simulink model "Symmetric"  (R2018a)
settings: Solver=VariableStepAuto  StartTime=0.0  StopTime=0.001  RelTol=1e-3
undefined symbols (not defined in the file or in its folder): fdesignblkfcn, G1, G2, G3, G4, G5, G6, G7, G8, gcbh, get, T
libraries: dspsrcs4 x1, dspxfrm3 x1, dspobslib x1
(part 1 of 2)
settings Model: Creator=Daniel  LastModifiedBy=Daniel

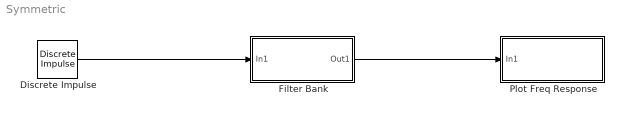
== system Symmetric ==
  Discrete Impulse : dspsrcs4/Discrete  Impulse  Delay=0  SampleTime=T  FrameSample=128  OutputFrames=off  dataType=double  isSigned=on  wordLen=16  udDataType=sfix(16)  fracBitsMode=Best precision  numFracBits=15  OutDataTypeStr=double  LastOutDataTypeStr=double
  "Filter Bank " : Subsystem
  Plot Freq Response : Subsystem
  wires:
  "Filter Bank "/1(Out1) -> Plot Freq Response/1(In1)
  Discrete Impulse/1 -> "Filter Bank "/1(In1)

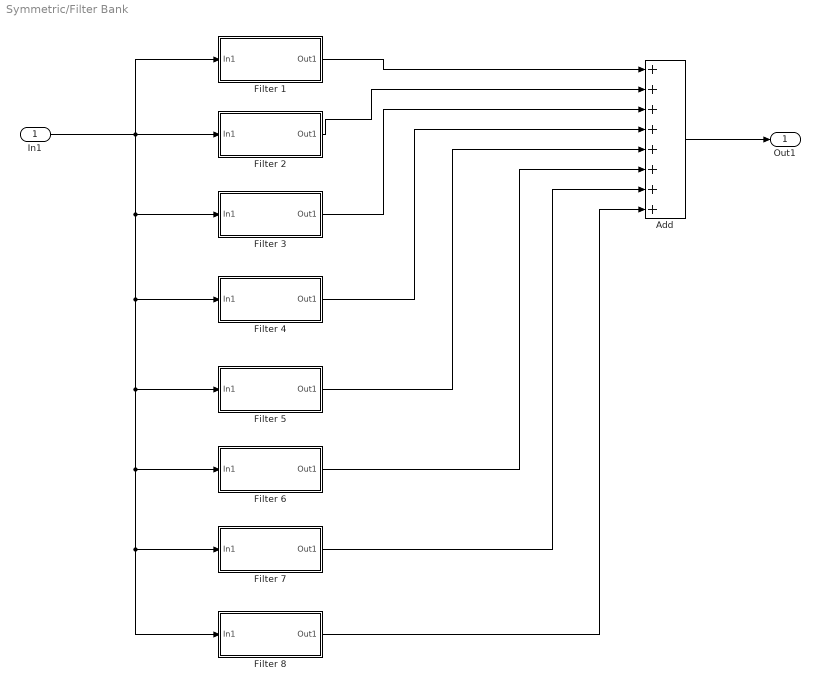
== system Symmetric/Filter Bank  ==
  In1 : Inport
  Add : Sum  Inputs=++++++++
  Filter 1 : Subsystem
  Filter 2 : Subsystem
  Filter 3 : Subsystem
  Filter 4 : Subsystem
  Filter 5 : Subsystem
  Filter 6 : Subsystem
  Filter 7 : Subsystem
  Filter 8 : Subsystem
  Out1 : Outport
  wires:
  In1/1 -> Filter 3/1(In1), Filter 6/1(In1), Filter 8/1(In1), Filter 7/1(In1), Filter 5/1(In1), Filter 4/1(In1), Filter 1/1(In1), Filter 2/1(In1)
  Add/1 -> Out1/1
  Filter 1/1(Out1) -> Add/1
  Filter 2/1(Out1) -> Add/2
  Filter 3/1(Out1) -> Add/3
  Filter 4/1(Out1) -> Add/4
  Filter 5/1(Out1) -> Add/5
  Filter 6/1(Out1) -> Add/6
  Filter 7/1(Out1) -> Add/7
  Filter 8/1(Out1) -> Add/8

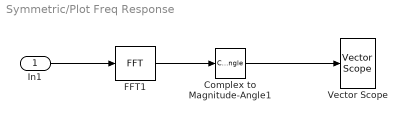
== system Symmetric/Plot Freq Response ==
  In1 : Inport
  Complex to Magnitude-Angle1 : ComplexToMagnitudeAngle  Output=Magnitude
  FFT1 : dspxfrm3/FFT  FFTImplementation=Auto  CompMethod=Table lookup  TableOpt=NEW  TableOptActive=Speed  BitRevOrder=off  Normalize=off  InheritFFTLength=on  FFTLength=64  WrapInput=on  roundingMode=Floor  overflowMode=off  firstCoeffDataTypeStr=Inherit: Same word length as input  firstCoeffLastDataTypeStr=Inherit: Same word length as input  outputMin=[]  outputMax=[]
  Vector Scope : dspobslib/Vector Scope  ScopeProperties=off  Domain=Frequency  HorizSpan=1  DisplayProperties=off  AxisGrid=on  Memory=off  FrameNumber=off  AxisLegend=off  AxisZoom=off  OpenScopeAtSimStart=on  OpenScopeImmediately=off  FigPos=get(0,'defaultfigureposition')  AxisProperties=on  XUnits=Hertz  XRange=[0...Fs/2]  InheritXIncr=on  XIncr=1  XLabel=Samples  XLimit=Auto  XMin=0  XMax=1  XStart=0  YUnits=dB  YLabel=|Magnitude (dB)|  LineProperties=off  XAxisParamsVer=6.9
      settings: SourceProductName=DSP System Toolbox  SourceProductBaseCode=DS  YMin=0.0723692553519949  YMax=69.3188381671759
  wires:
  In1/1 -> FFT1/1
  FFT1/1 -> Complex to Magnitude-Angle1/1
  Complex to Magnitude-Angle1/1 -> Vector Scope/1

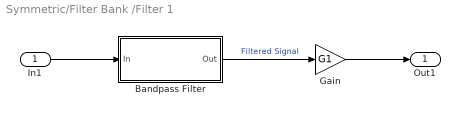
== system Symmetric/Filter Bank /Filter 1 ==
  In1 : Inport
  Bandpass Filter : Subsystem  DialogController=fdesignblkfcn  InitFcn=fdesignblkfcn(gcbh, {'InitFcn'});  mask(Bandpass Filter){}
      mask help: Design a bandpass filter
      settings: CopyFcn=fdesignblkfcn(gcbh, {'CopyFcn'});
      mask Help: helpview(mapfilelocation('dsp'), 'dspbandpassfilter');
      mask Display: disp('Bandpass');
  Gain : Gain  Gain=G1
  Out1 : Outport
  wires:
  Bandpass Filter/1(Out) -> Gain/1  "Filtered Signal"
  In1/1 -> Bandpass Filter/1(In)
  Gain/1 -> Out1/1

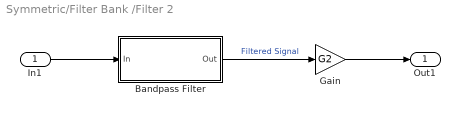
== system Symmetric/Filter Bank /Filter 2 ==
  In1 : Inport
  Bandpass Filter : Subsystem  DialogController=fdesignblkfcn  InitFcn=fdesignblkfcn(gcbh, {'InitFcn'});  mask(Bandpass Filter){}
      mask help: Design a bandpass filter
      settings: CopyFcn=fdesignblkfcn(gcbh, {'CopyFcn'});
      mask Help: helpview(mapfilelocation('dsp'), 'dspbandpassfilter');
      mask Display: disp('Bandpass');
  Gain : Gain  Gain=G2
  Out1 : Outport
  wires:
  Bandpass Filter/1(Out) -> Gain/1  "Filtered Signal"
  In1/1 -> Bandpass Filter/1(In)
  Gain/1 -> Out1/1

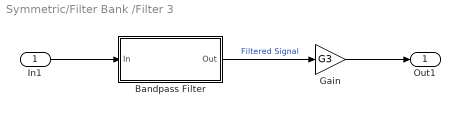
== system Symmetric/Filter Bank /Filter 3 ==
  In1 : Inport
  Bandpass Filter : Subsystem  DialogController=fdesignblkfcn  InitFcn=fdesignblkfcn(gcbh, {'InitFcn'});  mask(Bandpass Filter){}
      mask help: Design a bandpass filter
      settings: CopyFcn=fdesignblkfcn(gcbh, {'CopyFcn'});
      mask Help: helpview(mapfilelocation('dsp'), 'dspbandpassfilter');
      mask Display: disp('Bandpass');
  Gain : Gain  Gain=G3
  Out1 : Outport
  wires:
  Bandpass Filter/1(Out) -> Gain/1  "Filtered Signal"
  In1/1 -> Bandpass Filter/1(In)
  Gain/1 -> Out1/1

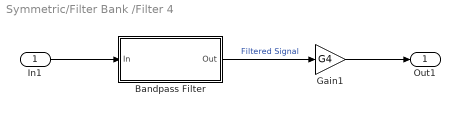
== system Symmetric/Filter Bank /Filter 4 ==
  In1 : Inport
  Bandpass Filter : Subsystem  DialogController=fdesignblkfcn  InitFcn=fdesignblkfcn(gcbh, {'InitFcn'});  mask(Bandpass Filter){}
      mask help: Design a bandpass filter
      settings: CopyFcn=fdesignblkfcn(gcbh, {'CopyFcn'});
      mask Help: helpview(mapfilelocation('dsp'), 'dspbandpassfilter');
      mask Display: disp('Bandpass');
  Gain1 : Gain  Gain=G4
  Out1 : Outport
  wires:
  Bandpass Filter/1(Out) -> Gain1/1  "Filtered Signal"
  In1/1 -> Bandpass Filter/1(In)
  Gain1/1 -> Out1/1

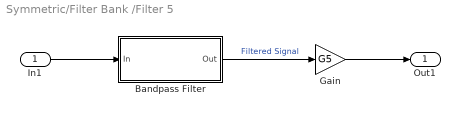
== system Symmetric/Filter Bank /Filter 5 ==
  In1 : Inport
  Bandpass Filter : Subsystem  DialogController=fdesignblkfcn  InitFcn=fdesignblkfcn(gcbh, {'InitFcn'});  mask(Bandpass Filter){}
      mask help: Design a bandpass filter
      settings: CopyFcn=fdesignblkfcn(gcbh, {'CopyFcn'});
      mask Help: helpview(mapfilelocation('dsp'), 'dspbandpassfilter');
      mask Display: disp('Bandpass');
  Gain : Gain  Gain=G5
  Out1 : Outport
  wires:
  Bandpass Filter/1(Out) -> Gain/1  "Filtered Signal"
  In1/1 -> Bandpass Filter/1(In)
  Gain/1 -> Out1/1

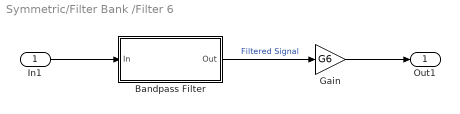
== system Symmetric/Filter Bank /Filter 6 ==
  In1 : Inport
  Bandpass Filter : Subsystem  DialogController=fdesignblkfcn  InitFcn=fdesignblkfcn(gcbh, {'InitFcn'});  mask(Bandpass Filter){}
      mask help: Design a bandpass filter
      settings: CopyFcn=fdesignblkfcn(gcbh, {'CopyFcn'});
      mask Help: helpview(mapfilelocation('dsp'), 'dspbandpassfilter');
      mask Display: disp('Bandpass');
  Gain : Gain  Gain=G6
  Out1 : Outport
  wires:
  Bandpass Filter/1(Out) -> Gain/1  "Filtered Signal"
  In1/1 -> Bandpass Filter/1(In)
  Gain/1 -> Out1/1

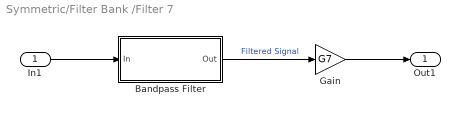
== system Symmetric/Filter Bank /Filter 7 ==
  In1 : Inport
  Bandpass Filter : Subsystem  DialogController=fdesignblkfcn  InitFcn=fdesignblkfcn(gcbh, {'InitFcn'});  mask(Bandpass Filter){}
      mask help: Design a bandpass filter
      settings: CopyFcn=fdesignblkfcn(gcbh, {'CopyFcn'});
      mask Help: helpview(mapfilelocation('dsp'), 'dspbandpassfilter');
      mask Display: disp('Bandpass');
  Gain : Gain  Gain=G7
  Out1 : Outport
  wires:
  Bandpass Filter/1(Out) -> Gain/1  "Filtered Signal"
  In1/1 -> Bandpass Filter/1(In)
  Gain/1 -> Out1/1

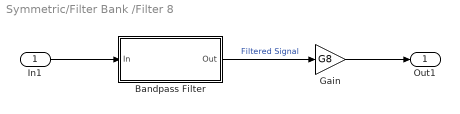
== system Symmetric/Filter Bank /Filter 8 ==
  In1 : Inport
  Bandpass Filter : Subsystem  DialogController=fdesignblkfcn  InitFcn=fdesignblkfcn(gcbh, {'InitFcn'});  mask(Bandpass Filter){}
      mask help: Design a bandpass filter
      settings: CopyFcn=fdesignblkfcn(gcbh, {'CopyFcn'});
      mask Help: helpview(mapfilelocation('dsp'), 'dspbandpassfilter');
      mask Display: disp('Bandpass');
  Gain : Gain  Gain=G8
  Out1 : Outport
  wires:
  Bandpass Filter/1(Out) -> Gain/1  "Filtered Signal"
  In1/1 -> Bandpass Filter/1(In)
  Gain/1 -> Out1/1

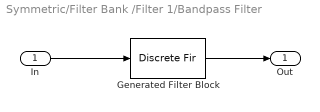
== system Symmetric/Filter Bank /Filter 1/Bandpass Filter ==
  In : Inport
  Generated Filter Block : DiscreteFir  Tag=BlockMethodSubSystem  Coefficients=[-0.288095935880251341 0.0525413418793297254 0.0469661528164785833 0.0413638961371985137 0.035743441875384814 0.0302610985045535484 0.0249161502944590801 0.0198560448668691492 0.0150617771881191003 0.010666253622455062 0.00662957256733126641 0.00307310029519767408 -7.12960758679805751e-05 -0.00269835686235154635 -0.00489597889786988483 -0.00657724977724275309 -0.00785309685969738311 -0.00864490861053823952 -0.00908979973506063472 -0.00911294285184072357 -0.00886997142217804853 -0.00828269872784345891 -0.00753185105272888202 -0.0065224375252314077 -0.0054576348610641005 -0.00422078667992279669 -0.00303593884382812084 -0.00174830873380574518 -0.000624644827463872749 0.000565354589150086689 0.00147289315421754116 0.00248164411845878258 0.00297649801950551803 0.00390644550655125378 0.00398986221425357869 0.00403163182400657384 0.00456913300373868771 0.00432952584417146263 0.00400413183887830121 0.00344452385152928036 0.00301759298676832367 0.0024648592619853733 0.00193704472346889608 0.00124269990373978298 0.000548146504904496691 -0.000233013280134805774 -0.000928086752325718274 -0.0016079036239721406 -0.00214342466057358509 -0.00261716452405418281 -0.00294642152557405852 -0.00321455590136646976 -0.00335513396218764222 -0.00343992999519496636 -0.00340818795304924848 -0.00331340319439810734 -0.00310534230123610776 -0.00283734411446902529 -0.0024686874963907833 -0.0020569757750758472 -0.00157932562542066851 -0.00108587602369365505 -0.00057464084255065865 -8.13931265320316902e-05 0.000379597218251630979 0.000803932237389910504 0.00116688807154375512 0.00140346382358171864 0.0017586610006951487 0.00174634027324323086 0.00186915640884384644 0.00190447992190369416 0.00184536222554758096 0.00164416184478038594 0.00144815028055871129 0.00120349413676317614 0.000953390304450837294 0.000615258083736531418 0.000258467885861202173 -0.000150488665692159111 -0.000520219390183063418 -0.000891696334957693291 -0.00120771657172187097 -0.00152010790567788136 -0.00177394667003233884 -0.00201259740633604042 -0.00217171226694658649 -0.00228852113553741935 -0.00230795208856010743 -0.00228053186210913725 -0.00215770975631921673 -0.00200597290924939579 -0.00178203504450490774 -0.00154713966436696108 -0.0012589304553587981 -0.000975184109959554841 -0.000647493809809341399 -0.000346389813347766965 -1.05485888533850436e-05 0.000256005081726213808 0.000577266056077218172 0.000756941456292188619 0.000985192320275318388 0.00113782558874355854 0.00118798764884436013 0.00123247243293567567 0.0012391642454049911 0.00116301132690384973 0.00103099208911635503 0.000863506020181792431 0.000681473816022045114 0.000453132507183181708 0.000193466705602888557 -0.000106363452799241865 -0.000406032554897162526 -0.000706800381284402863 -0.000984810227707108186 -0.00126094782477854201 -0.00150626261146827745 -0.00173150850840898709 -0.00190142474726660783 -0.00202931247623803742 -0.0020845945038517914 -0.00209873265242488871 -0.00204732530938491093 -0.00195812536072512014 -0.00181273083358852614 -0.00163528458599522986 -0.00140292268371900982 -0.00115138365696888963 -0.000853404855691656953 -0.000560408972579917513 -0.000237305797226729692 5.14958393311397135e-05 0.000346091011103256041 0.000621721693698512579 0.000829669047200214983 0.00105359212742192295 0.00120447865377228515 0.00129240756542236775 0.00134653604455318922 0.00134602513970211971 0.00127532081186506035 0.00113833590676117534 0.000964261511990258569 0.00074878023214015486 0.000496570402411653368 0.000204119261869774429 -0.000108583699207686528 -0.000434128584114584217 -0.000750409925752096568 -0.00106718699240494199 -0.00137092701931430219 -0.00166158721467703414 -0.00191329706170356413 -0.00212840560559363458 -0.00228636162366604306 -0.00239347382873119361 -0.00244426473573057003 -0.00244007154928103194 -0.00237105743965460025 -0.0022487583341873757 -0.00206062027136333457 -0.00182682342486109725 -0.00154175829205205513 -0.00122431695738080813 -0.00088053841024814854 -0.000509876951428265635 ...(+10068 chars)]  InputProcessing=Columns as channels (frame based)
  Out : Outport
  wires:
  In/1 -> Generated Filter Block/1
  Generated Filter Block/1 -> Out/1

== system Symmetric/Filter Bank /Filter 2/Bandpass Filter ==
  In : Inport
  Generated Filter Block : DiscreteFir  Tag=BlockMethodSubSystem  Coefficients=[0.0309918975999502432 -0.00346529452660930201 -0.00327768702863377726 -0.00308464127549961525 -0.00289652040207664246 -0.00268907563849799663 -0.00247512177193306981 -0.00223487476573661775 -0.00199009889114106636 -0.0017289884264930222 -0.0014863118531130079 -0.00125607889818925289 -0.00108386333736471691 -0.000960511740503544598 -0.000938888464479654961 -0.000986049090455784483 -0.00117022965780243932 -0.00143362593021634926 -0.00172184542701143972 -0.00217730583199699651 -0.00261066102832150509 -0.0030301462273852886 -0.00337634961355033972 -0.00363484969182988407 -0.00375610432847413994 -0.00372099799696547218 -0.00350134285661126213 -0.00309704321984028211 -0.00251514327490667822 -0.00178386307118819781 -0.0009453825375539196 -4.93028604005713023e-05 0.000835538086796441815 0.00166446108960707773 0.00235088687993217221 0.0028673032033801546 0.00318640123407974013 0.00324857894141917375 0.00308512556258552784 0.00270519389691393358 0.0021544847583524207 0.00147104446614270551 0.000722246214354252403 -3.31049707715524999e-05 -0.000723192415465159777 -0.00129554158302096212 -0.00170145006896672835 -0.0019183814855738418 -0.00193644757537291684 -0.00177079120537358692 -0.00145590729691326415 -0.00102883736774913442 -0.000563709798121668493 -0.000109919040585618188 0.000275905352650734903 0.000527180413109777646 0.000614396359583845031 0.000514639546278054805 0.000232848849020639292 -0.000216678184775262461 -0.000791226276756921976 -0.00144008427221523072 -0.00209286443000316486 -0.00268367262808864859 -0.00314258638437863586 -0.00341837730778005167 -0.00346705122035340096 -0.00327271796904423512 -0.00283815777153226256 -0.00218223382667261795 -0.00136120671786760933 -0.000429820163007577083 0.000541241331248352997 0.00147008604113440383 0.00228632324125550845 0.00292834038917961365 0.00335448506131175855 0.00353899144905925334 0.00348321369275839815 0.00320770011837738511 0.00275897358347381577 0.00219432073296702002 0.00158506057256413424 0.000996929500002817492 0.000498154064831682342 0.000135150835658563728 -5.88324711920454324e-05 -6.96927469107239128e-05 8.21939923249595528e-05 0.000364586300503982885 0.00072405344361104601 0.00109093618976985329 0.00139228754479791411 0.00155902633219394404 0.00153466511010429824 0.00127953804305375174 0.000778968397941552648 4.39103301674917401e-05 -0.000884542983329565657 -0.00194236596720676058 -0.00304340136920965704 -0.00409522039428792534 -0.00499532547765793589 -0.00565698977788660351 -0.00600465538531410117 -0.00598611782044648419 -0.00558681827129784217 -0.00482033314910380525 -0.00373427660887827237 -0.00240789823825553542 -0.00094343299551323534 0.000544322185675967518 0.00193832616447320999 0.00313008460357448379 0.00403005964624556304 0.00457683629750556611 0.00474436175826959197 0.00454465593503211238 0.00402744698218062899 0.00327073241174787727 0.00238272238628120525 0.00147720925602456282 0.000673387929664336082 7.91057236774334038e-05 -0.000226247434906512446 -0.000194578627544975125 0.000182554198220968855 0.000869879534658814235 0.00179136160269702943 0.0028376257945018149 0.00387609950437289852 0.0047643828925402025 0.00536388840592980434 0.00555577936429835564 0.00525368702911270871 0.00441732390407098899 0.00305707241014247996 0.00123383578647286163 -0.00093667086594187432 -0.00330373281024920473 -0.00568476798934752781 -0.00788433224413297856 -0.00971584946462498641 -0.0110163203016302481 -0.0116626099495929711 -0.0115862671070352113 -0.0107810443489587508 -0.00930520175755231507 -0.00727709012519854592 -0.00486507465144331297 -0.00227304784556266182 0.00027941037294022808 0.00257656143942119886 0.00443248056266570128 0.00570662954583686655 0.00631865065311489407 0.00626371902533782651 0.00560587550982431446 0.00448030932325531664 0.00307979850998303661 0.00163309043078356531 0.000383143549169649711 -0.000438246653694705779 -0.000638091039556747119 -8.5469583997715981e-05 0.00126893856190836429 0.00338196121334830013 0.00611453291286550085 ...(+5331 chars)]  InputProcessing=Columns as channels (frame based)
  Out : Outport
  wires:
  In/1 -> Generated Filter Block/1
  Generated Filter Block/1 -> Out/1

== system Symmetric/Filter Bank /Filter 3/Bandpass Filter ==
  In : Inport
  Generated Filter Block : DiscreteFir  Tag=BlockMethodSubSystem  Coefficients=[-0.0143532191975071794 0.0140053564122176229 0.00322487723732657605 -0.00341994842022029857 -0.00591206696740772739 -0.00507011043985050591 -0.0020869052544945782 0.00177518006656209038 0.00540121088137151054 0.00793552453768436167 0.00888969845469469305 0.0081749123586929949 0.00611628690310949893 0.00334148345787728396 0.000625906556626840832 -0.0013519514579631263 -0.00220138645705957731 -0.00194462863271905803 -0.000980757111720683555 6.09342188672840068e-05 0.000587506069177179402 0.00025782904804820192 -0.000847852852044458927 -0.00228848020789942236 -0.00337189109948501237 -0.00354293550486404693 -0.00243634794302895891 -0.000326790136062387465 0.00230028224699080006 0.00457585924112200587 0.00576530139547903539 0.0055616393876161685 0.00406190791969531992 0.00184589737010119881 -0.000243405106652175296 -0.00149619565701337651 -0.00161928339428159263 -0.00079351790775950351 0.000373340493504251136 0.0010807856607107022 0.000695133756775479644 -0.00092899593371771963 -0.00335277075515777456 -0.0057118706108804651 -0.00703374745259389977 -0.00660969492857268331 -0.00430747478209736814 -0.000665788661757951011 0.00324980883310138288 0.00625792298342621803 0.00747760285657104659 0.0067160320821627803 0.00446338026218173062 0.00177039526404422151 -0.000243772816674127368 -0.000806086259359652807 0.000178110254654275518 0.00202195663232857675 0.00358267146672195183 0.00370411846011775223 0.00174023051983389007 -0.00209407882997430378 -0.00673018371950949434 -0.0106262628634578478 -0.0123076296767781167 -0.0109571417722339193 -0.00678667980735296258 -0.00100338214019473487 0.00461379233822905785 0.00836205416977660668 0.00926630316427820913 0.00746394078237841777 0.0041666097883309855 0.00113900320645067207 -2.11036744678684551e-05 0.00139413487680974113 0.00486275050942145542 0.0087233865982068344 0.0108402564043355125 0.00945264485320536016 0.00399596996725636727 -0.00451758443571083704 -0.0137383669527115747 -0.0207282132149997633 -0.0230526346227897458 -0.0197382926529802265 -0.0117327832590544898 -0.00165349303776583106 0.00715052746451897911 0.0118870330536428453 0.0114437551594769454 0.00691804709851355504 0.00130370674297745556 -0.00167657593471810112 0.000862586529799574259 0.00956397285649513568 0.0221532285189574817 0.0338718040199820353 0.0389546484926311526 0.0327498677752619677 0.0136884438088064539 -0.0155454150015347011 -0.0482363721045643776 -0.0752668865467514686 -0.0878003964975626189 -0.0801238541990379194 -0.0517576845967735802 -0.00810391413228168239 0.0407304992780695707 0.0825886724476432577 0.106676497772512452 0.106676497772512452 0.0825886724476432577 0.0407304992780695707 -0.00810391413228168239 -0.0517576845967735802 -0.0801238541990379194 -0.0878003964975626189 -0.0752668865467514686 -0.0482363721045643776 -0.0155454150015347011 0.0136884438088064539 0.0327498677752619677 0.0389546484926311526 0.0338718040199820353 0.0221532285189574817 0.00956397285649513568 0.000862586529799574259 -0.00167657593471810112 0.00130370674297745556 0.00691804709851355504 0.0114437551594769454 0.0118870330536428453 0.00715052746451897911 -0.00165349303776583106 -0.0117327832590544898 -0.0197382926529802265 -0.0230526346227897458 -0.0207282132149997633 -0.0137383669527115747 -0.00451758443571083704 0.00399596996725636727 0.00945264485320536016 0.0108402564043355125 0.0087233865982068344 0.00486275050942145542 0.00139413487680974113 -2.11036744678684551e-05 0.00113900320645067207 0.0041666097883309855 0.00746394078237841777 0.00926630316427820913 0.00836205416977660668 0.00461379233822905785 -0.00100338214019473487 -0.00678667980735296258 -0.0109571417722339193 -0.0123076296767781167 -0.0106262628634578478 -0.00673018371950949434 -0.00209407882997430378 0.00174023051983389007 0.00370411846011775223 0.00358267146672195183 0.00202195663232857675 0.000178110254654275518 -0.000806086259359652807 -0.000243772816674127368 0.00177039526404422151 0.00446338026218173062 0.0067160320821627803 0.00747760285657104659 ...(+1178 chars)]  InputProcessing=Columns as channels (frame based)
  Out : Outport
  wires:
  In/1 -> Generated Filter Block/1
  Generated Filter Block/1 -> Out/1

== system Symmetric/Filter Bank /Filter 4/Bandpass Filter ==
  In : Inport
  Generated Filter Block : DiscreteFir  Tag=BlockMethodSubSystem  Coefficients=[0.0317027107068188971 0.00296912290738690372 -0.00273776081140421866 -0.00444938667259767075 -0.00173124240113138508 -0.00113663588381978189 -0.00585025491091577341 -0.00942768623505964125 -0.00424493210924422552 0.00658839504220370877 0.0114361670770268247 0.00522817453184396853 -0.00357354262483853798 -0.00453931373725491565 0.000145959474470844236 -0.000533231544595035847 -0.00918679538654094269 -0.0143588423242891772 -0.00614640338878158412 0.00846467016999057943 0.0135049248940609934 0.00556839029240450024 -0.00184764215889744797 0.00157068450479821227 0.00686718560861757869 -0.0011003591941983542 -0.0189069355947029567 -0.0249727303544332903 -0.00852077508232026819 0.0134894905523044398 0.0172163720783333647 0.00443490283705132247 -0.000445013017814264837 0.0123754838196375033 0.0203693718844136853 -0.000413253812070477902 -0.0357043495204128897 -0.0448210050961714013 -0.0143761880997315024 0.0195639997698436804 0.0186603099764099251 -0.00180556558244437644 0.0084542533270203675 0.0561532627627416153 0.0740808387472361024 -0.000761184138866498848 -0.126926244690189122 -0.174211416978599376 -0.0633127923736479109 0.126195730139845141 0.219518159767354948 0.126195730139845141 -0.0633127923736479109 -0.174211416978599376 -0.126926244690189122 -0.000761184138866498848 0.0740808387472361024 0.0561532627627416153 0.0084542533270203675 -0.00180556558244437644 0.0186603099764099251 0.0195639997698436804 -0.0143761880997315024 -0.0448210050961714013 -0.0357043495204128897 -0.000413253812070477902 0.0203693718844136853 0.0123754838196375033 -0.000445013017814264837 0.00443490283705132247 0.0172163720783333647 0.0134894905523044398 -0.00852077508232026819 -0.0249727303544332903 -0.0189069355947029567 -0.0011003591941983542 0.00686718560861757869 0.00157068450479821227 -0.00184764215889744797 0.00556839029240450024 0.0135049248940609934 0.00846467016999057943 -0.00614640338878158412 -0.0143588423242891772 -0.00918679538654094269 -0.000533231544595035847 0.000145959474470844236 -0.00453931373725491565 -0.00357354262483853798 0.00522817453184396853 0.0114361670770268247 0.00658839504220370877 -0.00424493210924422552 -0.00942768623505964125 -0.00585025491091577341 -0.00113663588381978189 -0.00173124240113138508 -0.00444938667259767075 -0.00273776081140421866 0.00296912290738690372 0.0317027107068188971]  InputProcessing=Columns as channels (frame based)
  Out : Outport
  wires:
  In/1 -> Generated Filter Block/1
  Generated Filter Block/1 -> Out/1

== system Symmetric/Filter Bank /Filter 5/Bandpass Filter ==
  In : Inport
  Generated Filter Block : DiscreteFir  Tag=BlockMethodSubSystem  Coefficients=[0.0326732231541482787 0.000390085683877424935 -0.00670927791321010176 0.000605921827593647625 0.00123859830126694655 0.000375200485484838487 0.00448384322372992819 0.000288098548715514898 -0.0108708572148590449 0.000561363559299206719 0.0113390583561961515 0.0004497822502392516 -0.00766228091096959624 0.000236985497879628471 -0.00213816414464076824 0.000485639836585969719 0.0109146397263644966 0.000493816262942203929 -0.0171652103124862593 0.000258137426842588156 0.0143757353938716737 0.000373935948854990392 -0.00542010433072735894 0.000532956822030185686 -0.009503867735852288 0.000303384827582722479 0.0212286144461720887 0.000279725809086309759 -0.0262814749571729338 0.000471320497063116857 0.0173994607544652007 0.000384902206955010917 0.00147013950558296013 0.000260885870586431972 -0.026407320499853601 0.000420059472173477642 0.0433997962924070266 0.000444031574083974428 -0.0442333827515434402 0.000284269280814331503 0.019081513210705451 0.000344216321775262792 0.028504282821260097 0.000450864822139246965 -0.0926582624495385226 0.000347618189527198194 0.155535524172606771 0.000295406621553085432 -0.203295061101749219 0.000410950165660755391 0.219908776572141612 0.000410950165660755391 -0.203295061101749219 0.000295406621553085432 0.155535524172606771 0.000347618189527198194 -0.0926582624495385226 0.000450864822139246965 0.028504282821260097 0.000344216321775262792 0.019081513210705451 0.000284269280814331503 -0.0442333827515434402 0.000444031574083974428 0.0433997962924070266 0.000420059472173477642 -0.026407320499853601 0.000260885870586431972 0.00147013950558296013 0.000384902206955010917 0.0173994607544652007 0.000471320497063116857 -0.0262814749571729338 0.000279725809086309759 0.0212286144461720887 0.000303384827582722479 -0.009503867735852288 0.000532956822030185686 -0.00542010433072735894 0.000373935948854990392 0.0143757353938716737 0.000258137426842588156 -0.0171652103124862593 0.000493816262942203929 0.0109146397263644966 0.000485639836585969719 -0.00213816414464076824 0.000236985497879628471 -0.00766228091096959624 0.0004497822502392516 0.0113390583561961515 0.000561363559299206719 -0.0108708572148590449 0.000288098548715514898 0.00448384322372992819 0.000375200485484838487 0.00123859830126694655 0.000605921827593647625 -0.00670927791321010176 0.000390085683877424935 0.0326732231541482787]  InputProcessing=Columns as channels (frame based)
  Out : Outport
  wires:
  In/1 -> Generated Filter Block/1
  Generated Filter Block/1 -> Out/1

== system Symmetric/Filter Bank /Filter 6/Bandpass Filter ==
  In : Inport
  Generated Filter Block : DiscreteFir  Tag=BlockMethodSubSystem  Coefficients=[-0.0299380034699614703 -0.00247053918462761604 0.00309964910196888072 -0.002911183051430212 0.00244203855890926663 -0.00278217532764521783 0.00331042991896847959 -0.00221217721175926037 -0.000282569252494490469 0.000989793467503130922 0.00220967307455731399 -0.00636592759066903924 0.00595651346285416133 -5.38432993041596149e-05 -0.00517507947373568519 0.00323203272160370054 0.00435094467552247198 -0.00888749592950219616 0.00512293740716600419 0.00269831226799241257 -0.00570881424568046771 0.00122421865229090489 0.0046915450541258983 -0.00543311403026824121 0.00167349353712737715 0.000991489886584623337 -0.000194343742086907148 -0.000912317391506925132 -0.000345954178242001767 0.00153434163851893374 0.000913842202165534093 -0.00511225150562856327 0.00507180157047438726 0.000809618685396407828 -0.00623743682841140096 0.00427603718139283641 0.00328145255578039287 -0.00767235627158433312 0.00407498278848102483 0.00259528822930395198 -0.00457257582826883779 0.00113190347045082768 0.00186757236464241833 -0.00117338190264310721 0.000235033296504368744 -0.00245890478467616913 0.00447317270177424731 -0.000708167273673825787 -0.00663031557414068065 0.00790564064003616493 0.00123030629567685151 -0.0115662581144963909 0.0101224217771004703 0.00302558858696458377 -0.0131742537470566148 0.00850839285061590934 0.0052097844076226061 -0.0120006030137155099 0.00554164000238210538 0.00436366768577950426 -0.00617967892152890969 0.00125826132512928124 0.000939370374617633924 0.00162711203993019804 -0.00106765755905567639 -0.00610303169124238112 0.0102415679503464752 -0.00126253392410721754 -0.0138517803149907394 0.0158669380864512807 0.00164565989441515376 -0.0202700661076546801 0.017309320845425441 0.00515891500974266504 -0.0213223956582095225 0.0133422040855330788 0.00705926020574866066 -0.0153607824307713803 0.00610813073122627725 0.00349719715551735644 -0.00142803831428164885 -0.00177925506859617083 -0.00731368872199610748 0.017990229565674417 -0.00606113466416884246 -0.0260982782520687573 0.0392668427789655827 -0.00399617769281149227 -0.0502907568474140199 0.0571336040755462404 0.00589416214014713835 -0.0757632001328289728 0.0674039989684223906 0.022068567165068026 -0.0969203312399510297 0.0674648890196974799 0.0410016481285865042 -0.108975533983563286 0.0576885876363833344 0.0576885876363833344 -0.108975533983563286 0.0410016481285865042 0.0674648890196974799 -0.0969203312399510297 0.022068567165068026 0.0674039989684223906 -0.0757632001328289728 0.00589416214014713835 0.0571336040755462404 -0.0502907568474140199 -0.00399617769281149227 0.0392668427789655827 -0.0260982782520687573 -0.00606113466416884246 0.017990229565674417 -0.00731368872199610748 -0.00177925506859617083 -0.00142803831428164885 0.00349719715551735644 0.00610813073122627725 -0.0153607824307713803 0.00705926020574866066 0.0133422040855330788 -0.0213223956582095225 0.00515891500974266504 0.017309320845425441 -0.0202700661076546801 0.00164565989441515376 0.0158669380864512807 -0.0138517803149907394 -0.00126253392410721754 0.0102415679503464752 -0.00610303169124238112 -0.00106765755905567639 0.00162711203993019804 0.000939370374617633924 0.00125826132512928124 -0.00617967892152890969 0.00436366768577950426 0.00554164000238210538 -0.0120006030137155099 0.0052097844076226061 0.00850839285061590934 -0.0131742537470566148 0.00302558858696458377 0.0101224217771004703 -0.0115662581144963909 0.00123030629567685151 0.00790564064003616493 -0.00663031557414068065 -0.000708167273673825787 0.00447317270177424731 -0.00245890478467616913 0.000235033296504368744 -0.00117338190264310721 0.00186757236464241833 0.00113190347045082768 -0.00457257582826883779 0.00259528822930395198 0.00407498278848102483 -0.00767235627158433312 0.00328145255578039287 0.00427603718139283641 -0.00623743682841140096 0.000809618685396407828 0.00507180157047438726 -0.00511225150562856327 0.000913842202165534093 0.00153434163851893374 -0.000345954178242001767 -0.000912317391506925132 -0.000194343742086907148 ...(+610 chars)]  InputProcessing=Columns as channels (frame based)
  Out : Outport
  wires:
  In/1 -> Generated Filter Block/1
  Generated Filter Block/1 -> Out/1
